simulink model "observer_sim"  (R2019b)
settings: Solver=ode4  StartTime=0.0  StopTime=40  FixedStep=0.01  RelTol=1e-3
values from neighbouring files (symbols this model uses):
  A = [0 1 0 0 ... (first row only)    [following.m]    (also in following2.m; observer.m; opt_servo.m; optimal_care.m = [0 1)
  B = [0 ... (first row only)    [following.m]    (also in following2.m; observer.m; opt_servo.m; optimal_care.m)
  C = [0 0 1 0]    [following.m]    (also in following2.m; observer.m; opt_servo.m)
  H = [-K 1]*inv(M0)*[zeros(4,1) ... (first row only)    [following.m]    (also in observer.m; optimal_hamilton.m = [A -B*inv(R)*B')
  K = -acker(A,B,p)    [following.m]    (also in following2.m = Ke(1:4); observer.m; opt_servo.m = -inv(Re)*B'*P11; optimal_care.m = -inv(R)*B'*P)
  L = -acker(A',C',q)'    [observer.m]
  x0 = zeros(4,1)    [following.m]    (also in following2.m; observer.m = [-0.5 0 0.5 0]'; opt_servo.m = [ 0 0 0.25 0 ]'; optimal_care.m = [1)
settings Model: Creator=shohei  LastModifiedBy=shohei

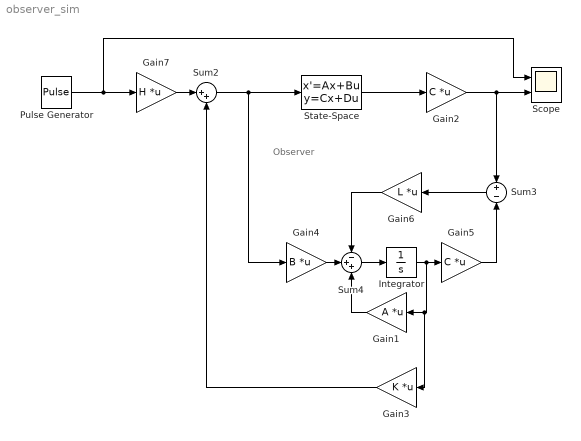
== system observer_sim ==
  note: Observer
  Gain1 : Gain  Gain=A  Multiplication=Matrix(K*u)
  Gain2 : Gain  Gain=C  Multiplication=Matrix(K*u)
  Gain3 : Gain  Gain=K  Multiplication=Matrix(K*u)
  Gain4 : Gain  Gain=B  Multiplication=Matrix(K*u)
  Gain5 : Gain  Gain=C  Multiplication=Matrix(K*u)
  Gain6 : Gain  Gain=L  Multiplication=Matrix(K*u)
  Gain7 : Gain  Gain=H  Multiplication=Matrix(K*u)
  Integrator : Integrator
  Pulse Generator : DiscretePulseGenerator  Period=10  PulseWidth=5  PhaseDelay=5
  Scope : Scope  NumInputPorts=2
  State-Space : StateSpace  A=A  B=B  C=eye(4)  D=zeros(4,1)  InitialCondition=x0
  Sum2 : Sum  Inputs=|++
  Sum3 : Sum  Inputs=+|-
  Sum4 : Sum  Inputs=-++
  wires:
  State-Space/1 -> Gain2/1
  Sum3/1 -> Gain6/1
  Gain5/1 -> Sum3/2
  Gain1/1 -> Sum4/3
  Sum4/1 -> Integrator/1
  Gain6/1 -> Sum4/1
  Gain4/1 -> Sum4/2
  Integrator/1 -> Gain3/1, Gain1/1, Gain5/1
  Gain2/1 -> Sum3/1, Scope/2
  Sum2/1 -> Gain4/1, State-Space/1
  Pulse Generator/1 -> Scope/1, Gain7/1
  Gain7/1 -> Sum2/1
  Gain3/1 -> Sum2/2
